simulink model "openLoopSystem"  (R2016a)
settings: Solver=ode45  StartTime=0.0  StopTime=10.0  RelTol=1e-3
values from neighbouring files (symbols this model uses):
  Gb = 200    [pole_placement.m]    (also in pole_placement2.m; time_domain.m)
  Ib = 0    [pole_placement.m]    (also in pole_placement2.m; time_domain.m)
  n = 0.142    [pole_placement.m]    (also in pole_placement2.m; time_domain.m)
  p1 = 0.035    [pole_placement.m]    (also in pole_placement2.m; time_domain.m)
  p2 = 0.05    [pole_placement.m]    (also in pole_placement2.m; time_domain.m)
  p3 = 0.000023    (= 2.3e-05)    [pole_placement.m]    (also in pole_placement2.m = 2.8e-05; time_domain.m)
  VG = 117    [pole_placement.m]    (also in pole_placement2.m; time_domain.m)
  VI = 1/0.098    (= 10.2040816327)    [pole_placement.m]    (also in pole_placement2.m; time_domain.m)
settings Model: Creator=joach  LastModifiedBy=User
settings DataIOCC: LimitDataPoints=on  SaveFormat=Array
settings DebuggingCC: SolverPrmCheckMsg=warning
settings HardwareCC: ProdBitPerPointer=32  ProdLargestAtomicFloat=None  ProdIntDivRoundTo=Undefined  ProdEndianess=Unspecified  ProdWordSize=32  ProdHWDeviceType=32-bit Generic
settings ModelReferenceCC: PropagateSignalLabelsOutOfModel=off
settings ConfigComp: CovModelRefEnable=Off  CovSFcnEnable=off

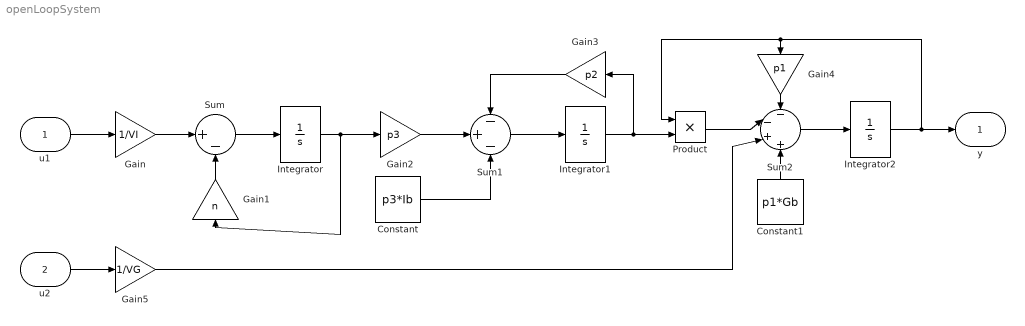
== system openLoopSystem ==
  u1 : Inport
  u2 : Inport  Port=2
  " Gain" : Gain  Gain=1/VI
  " Gain2" : Gain  Gain=p3
  " Gain3" : Gain  Gain=p2
  " Gain4" : Gain  Gain=p1
  " Gain5" : Gain  Gain=1/VG
  Constant : Constant  Value=p3*Ib
  Constant1 : Constant  Value=p1*Gb
  Gain1 : Gain  Gain=n
  Integrator : Integrator
  Integrator1 : Integrator
  Integrator2 : Integrator
  Product : Product
  Sum : Sum  Inputs=|+-
  Sum1 : Sum  Inputs=-+-
  Sum2 : Sum  Inputs=--++
  y : Outport
  wires:
  u1/1 -> " Gain"/1
  " Gain"/1 -> Sum/1
  Gain1/1 -> Sum/2
  Sum/1 -> Integrator/1
  Integrator/1 -> Gain1/1, " Gain2"/1
  " Gain2"/1 -> Sum1/2
  Constant/1 -> Sum1/3
  Sum1/1 -> Integrator1/1
  Product/1 -> Sum2/2
  Sum2/1 -> Integrator2/1
  Integrator2/1 -> y/1, " Gain4"/1, Product/1
  u2/1 -> " Gain5"/1
  " Gain5"/1 -> Sum2/3
  " Gain4"/1 -> Sum2/1
  Integrator1/1 -> " Gain3"/1, Product/2
  " Gain3"/1 -> Sum1/1
  Constant1/1 -> Sum2/4
